simulink model "q2section4"  (R2019a)
settings: Solver=VariableStepAuto  StartTime=0.0  StopTime=20  RelTol=1e-3
values from neighbouring files (symbols this model uses):
  g = 9.81    [q2.m]
  mL = 1000    [q2.m]
libraries: cstblocks x4
settings Model: Creator=Nir Lalum  LastModifiedBy=Nir Lalum

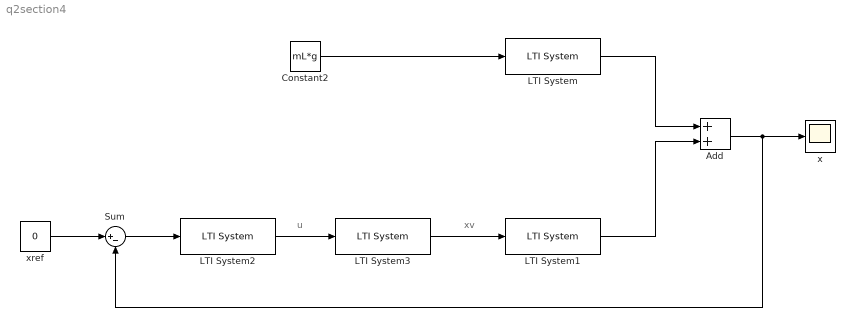
== system q2section4 ==
  note: u
  note: xv
  Add : Sum
  Constant2 : Constant  Value=mL*g
  LTI System : cstblocks/LTI System  sys=Pf  IC=[]
  LTI System1 : cstblocks/LTI System  sys=Pxv  IC=[]
  LTI System2 : cstblocks/LTI System  sys=Ctot  IC=[]
  LTI System3 : cstblocks/LTI System  sys=Pvalve  IC=[]
  Sum : Sum  Inputs=|+-
  "x " : Scope
  xref : Constant  Value=0
  wires:
  LTI System/1 -> Add/1
  Constant2/1 -> LTI System/1
  Add/1 -> Sum/2, "x "/1
  LTI System1/1 -> Add/2
  Sum/1 -> LTI System2/1
  xref/1 -> Sum/1
  LTI System2/1 -> LTI System3/1
  LTI System3/1 -> LTI System1/1
